simulink library "INP_EMRR"  (R2022a)
settings: Solver=VariableStepAuto  StartTime=0.0  StopTime=10.0  RelTol=1e-3
settings Model: Creator=blatak  LastModifiedBy=blatak

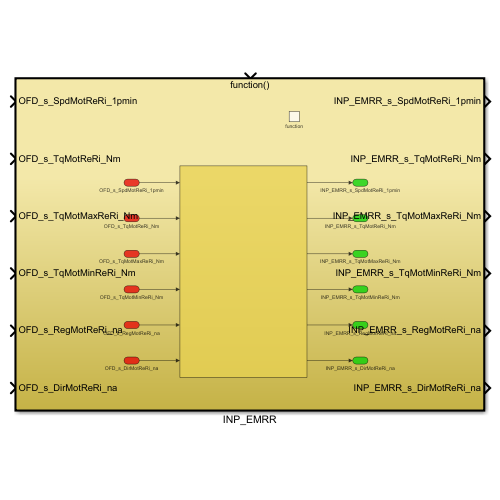
[thumbnail: Simulink's stored preview of the top-level diagram]
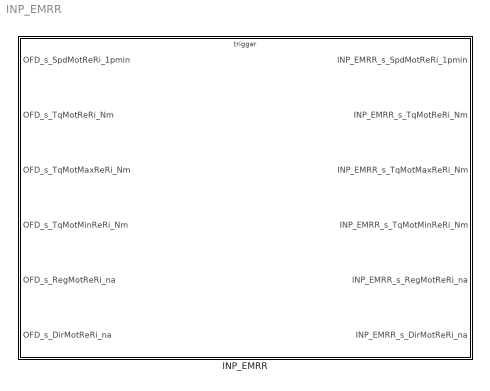
== system INP_EMRR ==
  INP_EMRR : Subsystem  TreatAsAtomicUnit=on

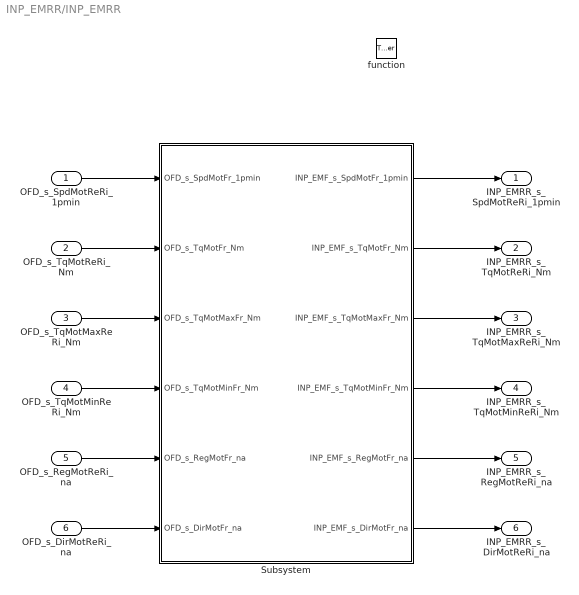
== system INP_EMRR/INP_EMRR ==
  OFD_s_SpdMotReRi_1pmin : Inport
  OFD_s_TqMotReRi_Nm : Inport  Port=2
  OFD_s_TqMotMaxReRi_Nm : Inport  Port=3
  OFD_s_TqMotMinReRi_Nm : Inport  Port=4
  OFD_s_RegMotReRi_na : Inport  Port=5
  OFD_s_DirMotReRi_na : Inport  Port=6
  function : TriggerPort  TriggerType=function-call  VariantControl=(inherit)
  Subsystem : Subsystem
  INP_EMRR_s_SpdMotReRi_1pmin : Outport
  INP_EMRR_s_TqMotReRi_Nm : Outport  Port=2
  INP_EMRR_s_TqMotMaxReRi_Nm : Outport  Port=3
  INP_EMRR_s_TqMotMinReRi_Nm : Outport  Port=4
  INP_EMRR_s_RegMotReRi_na : Outport  Port=5
  INP_EMRR_s_DirMotReRi_na : Outport  Port=6
  wires:
  OFD_s_TqMotReRi_Nm/1 -> Subsystem/2(OFD_s_TqMotFr_Nm)
  OFD_s_SpdMotReRi_1pmin/1 -> Subsystem/1(OFD_s_SpdMotFr_1pmin)
  Subsystem/1(INP_EMF_s_SpdMotFr_1pmin) -> INP_EMRR_s_SpdMotReRi_1pmin/1
  Subsystem/2(INP_EMF_s_TqMotFr_Nm) -> INP_EMRR_s_TqMotReRi_Nm/1
  OFD_s_TqMotMaxReRi_Nm/1 -> Subsystem/3(OFD_s_TqMotMaxFr_Nm)
  OFD_s_TqMotMinReRi_Nm/1 -> Subsystem/4(OFD_s_TqMotMinFr_Nm)
  OFD_s_RegMotReRi_na/1 -> Subsystem/5(OFD_s_RegMotFr_na)
  OFD_s_DirMotReRi_na/1 -> Subsystem/6(OFD_s_DirMotFr_na)
  Subsystem/3(INP_EMF_s_TqMotMaxFr_Nm) -> INP_EMRR_s_TqMotMaxReRi_Nm/1
  Subsystem/4(INP_EMF_s_TqMotMinFr_Nm) -> INP_EMRR_s_TqMotMinReRi_Nm/1
  Subsystem/5(INP_EMF_s_RegMotFr_na) -> INP_EMRR_s_RegMotReRi_na/1
  Subsystem/6(INP_EMF_s_DirMotFr_na) -> INP_EMRR_s_DirMotReRi_na/1

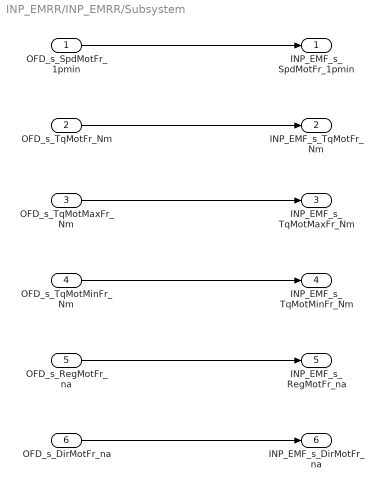
== system INP_EMRR/INP_EMRR/Subsystem ==
  OFD_s_SpdMotFr_1pmin : Inport
  OFD_s_TqMotFr_Nm : Inport  Port=2
  OFD_s_TqMotMaxFr_Nm : Inport  Port=3
  OFD_s_TqMotMinFr_Nm : Inport  Port=4
  OFD_s_RegMotFr_na : Inport  Port=5
  OFD_s_DirMotFr_na : Inport  Port=6
  INP_EMF_s_SpdMotFr_1pmin : Outport
  INP_EMF_s_TqMotFr_Nm : Outport  Port=2
  INP_EMF_s_TqMotMaxFr_Nm : Outport  Port=3
  INP_EMF_s_TqMotMinFr_Nm : Outport  Port=4
  INP_EMF_s_RegMotFr_na : Outport  Port=5
  INP_EMF_s_DirMotFr_na : Outport  Port=6
  wires:
  OFD_s_TqMotFr_Nm/1 -> INP_EMF_s_TqMotFr_Nm/1
  OFD_s_SpdMotFr_1pmin/1 -> INP_EMF_s_SpdMotFr_1pmin/1
  OFD_s_TqMotMaxFr_Nm/1 -> INP_EMF_s_TqMotMaxFr_Nm/1
  OFD_s_TqMotMinFr_Nm/1 -> INP_EMF_s_TqMotMinFr_Nm/1
  OFD_s_RegMotFr_na/1 -> INP_EMF_s_RegMotFr_na/1
  OFD_s_DirMotFr_na/1 -> INP_EMF_s_DirMotFr_na/1
